simulink subsystem "VL53L0"  (R2024b)
settings: Solver=VariableStepAuto  StartTime=0.0  StopTime=10.0  RelTol=1e-3
settings Model: Creator=JesseJabezArendse  LastModifiedBy=JesseJabezArendse

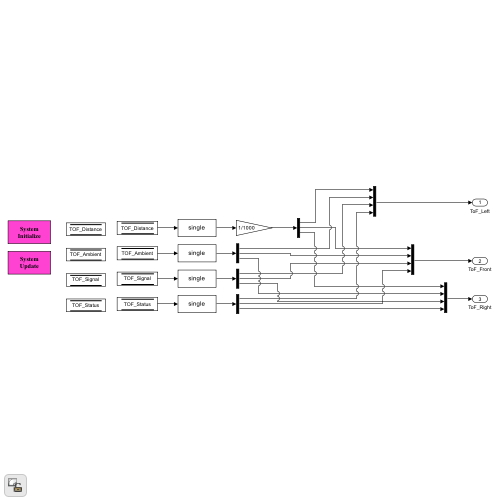
[thumbnail: Simulink's stored preview of the top-level diagram]
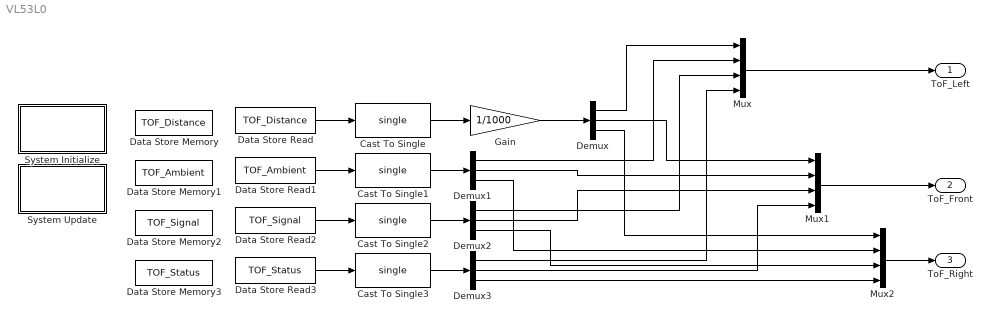
== system VL53L0 ==
  Cast To Single{,1..3} (4 alike) : DataTypeConversion  OutDataTypeStr=single  SaturateOnIntegerOverflow=off  RndMeth=Floor
  Data Store Memory : DataStoreMemory  DataStoreName=TOF_Distance  WriteAfterWriteMsg=warning  ShowAdditionalParam=off  OutDataTypeStr=uint32  Dimensions=3
  Data Store Memory1 : DataStoreMemory  DataStoreName=TOF_Ambient  WriteAfterWriteMsg=warning  ShowAdditionalParam=off  OutDataTypeStr=fixdt(1,9,7)  Dimensions=3
  Data Store Memory2 : DataStoreMemory  DataStoreName=TOF_Signal  WriteAfterWriteMsg=warning  ShowAdditionalParam=off  OutDataTypeStr=fixdt(1,9,7)  Dimensions=3
  Data Store Memory3 : DataStoreMemory  DataStoreName=TOF_Status  WriteAfterWriteMsg=warning  ShowAdditionalParam=off  OutDataTypeStr=uint32  Dimensions=3
  Data Store Read : DataStoreRead  DataStoreName=TOF_Distance  IndexOptions=Index vector (dialog)  Indices=1  OutputSizes=1
  Data Store Read1 : DataStoreRead  DataStoreName=TOF_Ambient  IndexOptions=Index vector (dialog)  Indices=1  OutputSizes=1
  Data Store Read2 : DataStoreRead  DataStoreName=TOF_Signal  IndexOptions=Index vector (dialog)  Indices=1  OutputSizes=1
  Data Store Read3 : DataStoreRead  DataStoreName=TOF_Status  IndexOptions=Index vector (dialog)  Indices=1  OutputSizes=1
  Demux{,1..3} (4 alike) : Demux  Outputs=3
  Gain : Gain  Gain=1/1000
  Mux : Mux
  Mux1 : Mux
  Mux2 : Mux
  System Initialize : Subsystem  mask(System Initialize){ShowInLibBrowser=0}
      mask prompts: ShowInLibBrowser "Simulink:masks:CustCodeMaskParam1_MP"
      settings: CopyFcn=cccopyfcn(gcb)  OpenFcn=ccopenfcn('System Initialize Function')
      mask Help: eval('feval(''rtwprivate'',''rtwhelpview'',''rtw_sys_initialize_block'')');
      mask Display: disp('System\nInitialize');
  System Update : Subsystem  mask(System Update){ShowInLibBrowser=0}
      mask prompts: ShowInLibBrowser "Simulink:masks:CustCodeMaskParam1_MP"
      settings: CopyFcn=cccopyfcn(gcb)  OpenFcn=ccopenfcn('System Update Function')
      mask Help: eval('feval(''rtwprivate'',''rtwhelpview'',''rtw_sys_update_block'')');
      mask Display: disp('System\nUpdate');
  ToF_Left : Outport  OutDataTypeStr=single  PortDimensions=4
  ToF_Front : Outport  Port=2  OutDataTypeStr=single  PortDimensions=4
  ToF_Right : Outport  Port=3  OutDataTypeStr=single  PortDimensions=4
  wires:
  Data Store Read/1 -> Cast To Single/1
  Cast To Single/1 -> Gain/1
  Cast To Single1/1 -> Demux1/1
  Data Store Read1/1 -> Cast To Single1/1
  Cast To Single2/1 -> Demux2/1
  Data Store Read2/1 -> Cast To Single2/1
  Cast To Single3/1 -> Demux3/1
  Data Store Read3/1 -> Cast To Single3/1
  Gain/1 -> Demux/1
  Demux/1 -> Mux/1
  Demux1/1 -> Mux/2
  Demux2/1 -> Mux/3
  Demux3/1 -> Mux/4
  Demux/2 -> Mux1/1
  Demux1/2 -> Mux1/2
  Demux2/2 -> Mux1/3
  Demux3/2 -> Mux1/4
  Demux/3 -> Mux2/1
  Demux1/3 -> Mux2/2
  Demux2/3 -> Mux2/3
  Demux3/3 -> Mux2/4
  Mux/1 -> ToF_Left/1
  Mux1/1 -> ToF_Front/1
  Mux2/1 -> ToF_Right/1

== system VL53L0/System Initialize ==

== system VL53L0/System Update ==
